simulink model "atrias_nmm_hardware"  (R2014b)
settings: Solver=ode4  StartTime=0.0  StopTime=inf  FixedStep=sample_time  RelTol=1e-3
undefined symbols (not defined in the file): A_lpf_dtau, B1_lpf_dtau, B2_lpf_dtau, boom_mount_angle, boom_pelvis_offset_angle, c, c_jointstop, contactThr, control_start_time, D12_T, d_y_boom_com_offset, d_y_boom_hip_offset, eref, fcut_contact, FmaxBFSH, FmaxGLU, FmaxHAM, FmaxHFL, FmaxRF, FmaxVAS, g, h_boom, HIP_MTR_MAX_CONT_TORQUE, initial_com_height, initial_dx, K, k_sea, kd_lateral, kd_phi12, kd_phi23, kp_lateral, kp_phi12, kp_phi23, l_boom_projected, L_distribution_switch, L_force_ctrl_switch, L_hip_trq_desired, L_knee_trq_desired, L_sea_input_switch, l_seg, L_stim_gain, L_stim_switch, l_yaw_center_to_pelvis, lambdaHip, lambdaKnee, lateral_offset, lateral_target_angle_left, lateral_target_angle_right, lateral_transition_force, loptBFSH, loptGLU, loptHAM, loptHFL, loptRF, loptVAS, Lphi12_des, Lphi23_des, lslackBFSH, lslackGLU, lslackHAM ... (+69)
libraries: simulink_extras x15, simulink x5, slrtlib x3
(part 2 of 9)

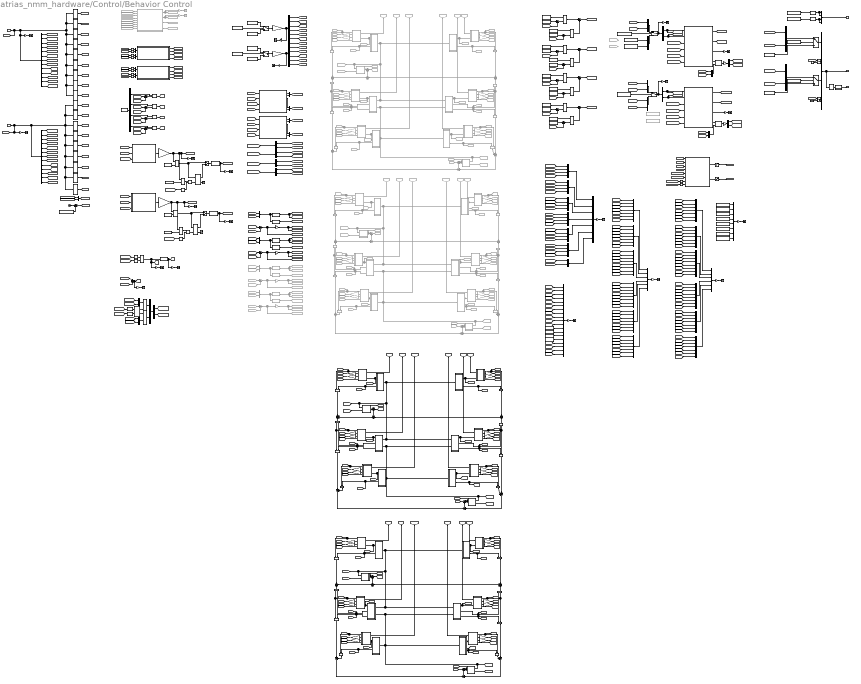
== system atrias_nmm_hardware/Control/Behavior Control ==
  note: Velocity Estimation
  note: Muscle Stimulation Input
  note: Leg/Spring Measurements
  note: Lateral Behavior
  note: Torque Commands
  note: Inputs
  note: q Order:
      |
      | backJointR
      | backGearR
      | frontJointR
      | frontGearR
      |
      | backJointL
      | backGearL
      | frontJointL
      | frontGearL
      |
      | latR
      | latL
      |
      | boomRoll
      | boomYaw
      | boomPitch
  note: Motor Order:
      |
      | backR
      | frontR
      | latR
      | backL
      | frontL
      | latL
  note: Muscle Geometry Input
  note: Atrias Knee/Splay Angles
  note: Estimate SEA Torque
  note: Estimate Leg Load and Contact
  note: Hip/Knee Torque Distribution
  note: Left Leg
  note: Neural Control Layer Interface
  note: Discrete Muscle Actuation Layer
  note: Body Mechanics Layer
      | Interface (Left Hip Joint)
  note: Body Mechanics Layer
      | Interface (Left Knee Joint)
  note: Right Leg
  note: Neural Control Layer Interface
  note: Body Mechanics Layer
      | Interface (Left Hip Joint)
  note: Body Mechanics Layer
      | Interface (Left Knee Joint)
  note: Estimate Flight/Escape
  note: Estimate GRFy
  note: Estimate Primary Leg Length/Angle
  note: Position Control
  note: Export Data
  note: Left Leg
  note: Neural Control Layer Interface
  note: Continuous Muscle Actuation Layer
  note: Body Mechanics Layer
      | Interface (Left Hip Joint)
  note: Body Mechanics Layer
      | Interface (Left Knee Joint)
  note: Right Leg
  note: Neural Control Layer Interface
  note: Body Mechanics Layer
      | Interface (Left Hip Joint)
  note: Body Mechanics Layer
      | Interface (Left Knee Joint)
  dq_cmu : Inport
  q_cmu : Inport  Port=2
  Clock : Clock
  Constant{,1,26,30,34,38} (6 alike) : Constant  Value=0
  Constant10 : Constant  Value=releaseThr
  Constant11 : Constant  Value=contactThr
  Constant12 : Constant  Value=releaseThr
  Constant13 : Constant  Commented=on  Value=L_knee_trq_desired
  Constant14 : Constant  Value=R_knee_trq_desired
  Constant15 : Constant  Value=R_distribution_switch
  Constant16 : Constant  Value=L_distribution_switch
  Constant17 : Constant  Value=R_sea_input_switch
  Constant18 : Constant  Value=L_sea_input_switch
  Constant19 : Constant  Value=[0;0]
  Constant2 : Constant  Value=control_start_time
  Constant20 : Constant  Value=[0;0]
  Constant21 : Constant  Value=R_hip_trq_desired
  Constant22 : Constant  Commented=on  Value=L_hip_trq_desired
  Constant23 : Constant  Value=k_sea
  Constant24 : Constant  Value=Lphi12_des
  Constant25 : Constant  Value=kp_phi12
  Constant27 : Constant  Value=kd_phi12
  Constant28 : Constant  Value=Lphi23_des
  Constant29 : Constant  Value=kp_phi23
  Constant3 : Constant  Value=LStim_Constant
  Constant31 : Constant  Value=kd_phi23
  Constant32 : Constant  Value=Rphi12_des
  Constant33 : Constant  Value=kp_phi12
  Constant35 : Constant  Value=kd_phi12
  Constant36 : Constant  Value=Rphi23_des
  Constant37 : Constant  Value=kp_phi23
  Constant39 : Constant  Value=kd_phi23
  Constant4 : Constant  Value=RStim_Constant
  Constant40 : Constant  Value=Lphi23_des
  Constant41 : Constant  Value=Lphi12_des
  Constant42 : Constant  Value=Rphi23_des
  Constant43 : Constant  Value=Rphi12_des
  Constant44 : Constant  Value=R_force_ctrl_switch
  Constant45 : Constant  Value=L_force_ctrl_switch
  Constant46 : Constant  Value=R_distribution_switch
  Constant47 : Constant  Value=L_distribution_switch
  Constant48 : Constant  Value=R_stim_switch
  Constant49 : Constant  Value=L_stim_switch
  Constant5 : Constant  Value=[0;0;0;0;0;0]
  Constant50 : Constant  Value=R_force_ctrl_switch
  Constant51 : Constant  Value=L_force_ctrl_switch
  Constant52 : Constant  Value=R_sea_input_switch
  Constant53 : Constant  Value=L_sea_input_switch
  Constant6 : Constant  Value=[0;0;0;0;0;0]
  Constant7 : Constant  Value=R_stim_switch
  Constant8 : Constant  Value=L_stim_switch
  Constant9 : Constant  Value=contactThr
  Data Type Conversion : DataTypeConversion  OutDataTypeStr=double
  Data Type Conversion1 : DataTypeConversion  OutDataTypeStr=double
  Data Type Conversion{2..5} (4 alike) : DataTypeConversion  OutDataTypeStr=boolean
  Demux{,1,3,14..19} (9 alike) : Demux  Outputs=2
  Demux11 : Demux  Outputs=6
  Demux12 : Demux  Outputs=13
  Demux13 : Demux  Outputs=13
  Demux2 : Demux  Outputs=6
  Demux4 : Demux
  Detect Increase : simulink/Logic and Bit Operations/Detect Increase  vinit=0.0  InputProcessing=Inherited  OutDataTypeStr=boolean
  From10 : From  Commented=on  GotoTag=Lphi12  TagVisibility=global
      settings: CloseFcn=tagdialog Close
  From116 : From  Commented=on  GotoTag=qBoomYaw
  From12 : From  Commented=on  GotoTag=Ldphi23  TagVisibility=global
      settings: CloseFcn=tagdialog Close
  From13 : From  Commented=on  GotoTag=RStimVAS  TagVisibility=global
      settings: CloseFcn=tagdialog Close
  From16 : From  Commented=on  GotoTag=Rdphi23  TagVisibility=global
      settings: CloseFcn=tagdialog Close
  From17 : From  Commented=on  GotoTag=Lphi23  TagVisibility=global
      settings: CloseFcn=tagdialog Close
  From19 : From  Commented=on  GotoTag=RStimRF  TagVisibility=global
      settings: CloseFcn=tagdialog Close
  From21 : From  Commented=on  GotoTag=LStimRF  TagVisibility=global
      settings: CloseFcn=tagdialog Close
  From22 : From  Commented=on  GotoTag=GRFy
  From23 : From  Commented=on  GotoTag=RStimHAM  TagVisibility=global
      settings: CloseFcn=tagdialog Close
  From24 : From  Commented=on  GotoTag=Ldphi12  TagVisibility=global
      settings: CloseFcn=tagdialog Close
  From25 : From  Commented=on  GotoTag=RStimHFL  TagVisibility=global
      settings: CloseFcn=tagdialog Close
  From26 : From  Commented=on  GotoTag=RStimGLU  TagVisibility=global
      settings: CloseFcn=tagdialog Close
  From260 : From  Commented=on  GotoTag=Lphi_thigh  TagVisibility=global
  From261 : From  Commented=on  GotoTag=Lphi_shin  TagVisibility=global
  From262 : From  Commented=on  GotoTag=Ldphi_thigh  TagVisibility=global
  From263 : From  Commented=on  GotoTag=Rphi_thigh  TagVisibility=global
  From264 : From  Commented=on  GotoTag=Rphi_shin  TagVisibility=global
  From265 : From  Commented=on  GotoTag=Rdphi_thigh  TagVisibility=global
  From266 : From  Commented=on  GotoTag=Rdphi_shin  TagVisibility=global
  From267 : From  Commented=on  GotoTag=Ldphi_shin  TagVisibility=global
  From28 : From  Commented=on  GotoTag=dqBoomYaw
  From29 : From  Commented=on  GotoTag=qBoomRoll
  From33 : From  Commented=on  GotoTag=RStimBFSH  TagVisibility=global
      settings: CloseFcn=tagdialog Close
  From34 : From  Commented=on  GotoTag=Rphi12  TagVisibility=global
      settings: CloseFcn=tagdialog Close
  From35 : From  Commented=on  GotoTag=LStimHAM  TagVisibility=global
      settings: CloseFcn=tagdialog Close
  From36 : From  Commented=on  GotoTag=Rdphi12  TagVisibility=global
      settings: CloseFcn=tagdialog Close
  From37 : From  Commented=on  GotoTag=LStimHFL  TagVisibility=global
      settings: CloseFcn=tagdialog Close
  From38 : From  Commented=on  GotoTag=LStimGLU  TagVisibility=global
      settings: CloseFcn=tagdialog Close
  From39 : From  Commented=on  GotoTag=LStimBFSH  TagVisibility=global
      settings: CloseFcn=tagdialog Close
  From40 : From  Commented=on  GotoTag=Rphi23  TagVisibility=global
      settings: CloseFcn=tagdialog Close
  From45 : From  Commented=on  GotoTag=TorsoPitch
  From50 : From  Commented=on  GotoTag=PrimaryLegAngle
  From51 : From  Commented=on  GotoTag=PrimaryLegLength
  From52 : From  Commented=on  GotoTag=dqBoomRoll
  From69 : From  Commented=on  GotoTag=RM23_pd  TagVisibility=global
  From70 : From  Commented=on  GotoTag=RM12_pd  TagVisibility=global
  From81 : From  Commented=on  GotoTag=escape
  From9 : From  Commented=on  GotoTag=LStimVAS  TagVisibility=global
      settings: CloseFcn=tagdialog Close
  GLU : Subsystem
  GLU Link : Subsystem  Commented=on
  GLU Link1 : Subsystem  Commented=on
  GLU Link2 : Subsystem
  GLU Link3 : Subsystem
  GLU1 : Subsystem
  GRFy : Gain
  Gain{,2,4..5} (4 alike) : Gain  Gain=-1
  Gain1 : Gain  Gain=R_stim_gain
  Gain3 : Gain  Gain=L_stim_gain
  Gain6 : Gain  Commented=on  Gain=-1
  Gain7 : Gain  Commented=on  Gain=-1
  Goto100 : Goto  Commented=on  GotoTag=RHipStop  TagVisibility=global
  Goto101 : Goto  Commented=on  GotoTag=RKneeStop  TagVisibility=global
  Goto102 : Goto  Commented=on  GotoTag=RLceHFL  TagVisibility=global
  Goto103 : Goto  Commented=on  GotoTag=RActRF  TagVisibility=global
  Goto104 : Goto  Commented=on  GotoTag=LFmRF  TagVisibility=global
  Goto105 : Goto  Commented=on  GotoTag=RActBFSH  TagVisibility=global
  Goto106 : Goto  Commented=on  GotoTag=RActVAS  TagVisibility=global
  Goto107 : Goto  Commented=on  GotoTag=RVceHAM  TagVisibility=global
  Goto108 : Goto  Commented=on  GotoTag=RrBFSH  TagVisibility=global
  Goto109 : Goto  Commented=on  GotoTag=RVceGLU  TagVisibility=global
  Goto110 : Goto  Commented=on  GotoTag=RLceGLU  TagVisibility=global
  Goto111 : Goto  Commented=on  GotoTag=RFmHFL  TagVisibility=global
  Goto112 : Goto  Commented=on  GotoTag=RVceVAS  TagVisibility=global
  Goto113 : Goto  Commented=on  GotoTag=LHipStop  TagVisibility=global
  Goto114 : Goto  Commented=on  GotoTag=LKneeStop  TagVisibility=global
  Goto115 : Goto  Commented=on  GotoTag=LLmtuBFSH  TagVisibility=global
  Goto116 : Goto  Commented=on  GotoTag=LActRF  TagVisibility=global
  Goto117 : Goto  Commented=on  GotoTag=LActBFSH  TagVisibility=global
  Goto124 : Goto  Commented=on  GotoTag=LFmBFSH  TagVisibility=global
  Goto126 : Goto  Commented=on  GotoTag=LVceHFL  TagVisibility=global
  Goto133 : Goto  Commented=on  GotoTag=Lphi_lower_splay  TagVisibility=global
  Goto134 : Goto  Commented=on  GotoTag=Ldphi_lower_splay  TagVisibility=global
  Goto135 : Goto  Commented=on  GotoTag=Lphi_back_knee  TagVisibility=global
  Goto136 : Goto  Commented=on  GotoTag=Ldphi_back_knee  TagVisibility=global
  Goto137 : Goto  Commented=on  GotoTag=Lphi_front_knee  TagVisibility=global
  Goto138 : Goto  Commented=on  GotoTag=Ldphi_front_knee  TagVisibility=global
  Goto139 : Goto  Commented=on  GotoTag=Rphi_lower_splay  TagVisibility=global
  Goto140 : Goto  Commented=on  GotoTag=Rdphi_lower_splay  TagVisibility=global
  Goto141 : Goto  Commented=on  GotoTag=Rphi_back_knee  TagVisibility=global
  Goto142 : Goto  Commented=on  GotoTag=Rdphi_back_knee  TagVisibility=global
  Goto143 : Goto  Commented=on  GotoTag=Rphi_front_knee  TagVisibility=global
  Goto144 : Goto  Commented=on  GotoTag=Rdphi_front_knee  TagVisibility=global
  Goto22 : Goto  Commented=on  GotoTag=LM12  TagVisibility=global
  Goto23 : Goto  Commented=on  GotoTag=RM12  TagVisibility=global
  Goto24 : Goto  Commented=on  GotoTag=LM23  TagVisibility=global
  Goto26 : Goto  Commented=on  GotoTag=dx_avg
  Goto27 : Goto  Commented=on  GotoTag=LLmtuVAS  TagVisibility=global
  Goto28 : Goto  Commented=on  GotoTag=RFmRF  TagVisibility=global
  Goto36 : Goto  Commented=on  GotoTag=LrHFL  TagVisibility=global
  Goto37 : Goto  Commented=on  GotoTag=LActHAM  TagVisibility=global
  Goto38 : Goto  Commented=on  GotoTag=LActGLU  TagVisibility=global
  Goto39 : Goto  Commented=on  GotoTag=LActHFL  TagVisibility=global
  Goto40 : Goto  Commented=on  GotoTag=LrHAMh  TagVisibility=global
  Goto41 : Goto  Commented=on  GotoTag=LrHAMk  TagVisibility=global
  Goto42 : Goto  Commented=on  GotoTag=LLceHAM  TagVisibility=global
  Goto43 : Goto  Commented=on  GotoTag=LrRFh  TagVisibility=global
  Goto44 : Goto  Commented=on  GotoTag=LrRFk  TagVisibility=global
  Goto45 : Goto  Commented=on  GotoTag=LLmtuRF  TagVisibility=global
  Goto46 : Goto  Commented=on  GotoTag=LrVAS  TagVisibility=global
  Goto47 : Goto  Commented=on  GotoTag=LLceRF  TagVisibility=global
  Goto48 : Goto  Commented=on  GotoTag=dy_avg
  Goto49 : Goto  Commented=on  GotoTag=tApex
  Goto50 : Goto  Commented=on  GotoTag=systemEnergy
  Goto51 : Goto  Commented=on  GotoTag=LVceBFSH  TagVisibility=global
  Goto52 : Goto  Commented=on  GotoTag=LLceBFSH  TagVisibility=global
  Goto53 : Goto  Commented=on  GotoTag=LLceVAS  TagVisibility=global
  Goto54 : Goto  Commented=on  GotoTag=LLmtuHFL  TagVisibility=global
  Goto56 : Goto  Commented=on  GotoTag=LFmGLU  TagVisibility=global
  Goto57 : Goto  Commented=on  GotoTag=LVceRF  TagVisibility=global
  Goto58 : Goto  Commented=on  GotoTag=LFmHAM  TagVisibility=global
  Goto59 : Goto  Commented=on  GotoTag=LFmVAS  TagVisibility=global
  Goto60 : Goto  Commented=on  GotoTag=RLmtuGLU  TagVisibility=global
  Goto61 : Goto  Commented=on  GotoTag=RLmtuHAM  TagVisibility=global
  Goto62 : Goto  Commented=on  GotoTag=LrGLU  TagVisibility=global
  Goto63 : Goto  Commented=on  GotoTag=RM23  TagVisibility=global
  Goto64 : Goto  Commented=on  GotoTag=RLmtuBFSH  TagVisibility=global
  Goto65 : Goto  Commented=on  GotoTag=RLmtuVAS  TagVisibility=global
  Goto66 : Goto  Commented=on  GotoTag=LLceHFL  TagVisibility=global
  Goto67 : Goto  Commented=on  GotoTag=RLmtuRF  TagVisibility=global
  Goto68 : Goto  Commented=on  GotoTag=LActVAS  TagVisibility=global
  Goto69 : Goto  Commented=on  GotoTag=LVceHAM  TagVisibility=global
  Goto70 : Goto  Commented=on  GotoTag=RFmBFSH  TagVisibility=global
  Goto71 : Goto  Commented=on  GotoTag=RVceHFL  TagVisibility=global
  Goto72 : Goto  Commented=on  GotoTag=RrHFL  TagVisibility=global
  Goto73 : Goto  Commented=on  GotoTag=RActHAM  TagVisibility=global
  Goto74 : Goto  Commented=on  GotoTag=RLmtuHFL  TagVisibility=global
  Goto75 : Goto  Commented=on  GotoTag=RActGLU  TagVisibility=global
  Goto76 : Goto  Commented=on  GotoTag=RActHFL  TagVisibility=global
  Goto77 : Goto  Commented=on  GotoTag=RrHAMh  TagVisibility=global
  Goto79 : Goto  Commented=on  GotoTag=RrHAMk  TagVisibility=global
  Goto80 : Goto  Commented=on  GotoTag=LLmtuGLU  TagVisibility=global
  Goto81 : Goto  Commented=on  GotoTag=RLceHAM  TagVisibility=global
  Goto82 : Goto  Commented=on  GotoTag=RrRFh  TagVisibility=global
  Goto83 : Goto  Commented=on  GotoTag=RrRFk  TagVisibility=global
  Goto84 : Goto  Commented=on  GotoTag=RrVAS  TagVisibility=global
  Goto85 : Goto  Commented=on  GotoTag=RLceRF  TagVisibility=global
  Goto86 : Goto  Commented=on  GotoTag=LVceGLU  TagVisibility=global
  Goto87 : Goto  Commented=on  GotoTag=LLceGLU  TagVisibility=global
  Goto88 : Goto  Commented=on  GotoTag=LFmHFL  TagVisibility=global
  Goto89 : Goto  Commented=on  GotoTag=RVceBFSH  TagVisibility=global
  Goto90 : Goto  Commented=on  GotoTag=LLmtuHAM  TagVisibility=global
  Goto91 : Goto  Commented=on  GotoTag=RLceBFSH  TagVisibility=global
  Goto92 : Goto  Commented=on  GotoTag=RLceVAS  TagVisibility=global
  Goto93 : Goto  Commented=on  GotoTag=LVceVAS  TagVisibility=global
  Goto94 : Goto  Commented=on  GotoTag=RFmGLU  TagVisibility=global
  Goto95 : Goto  Commented=on  GotoTag=RVceRF  TagVisibility=global
  Goto96 : Goto  Commented=on  GotoTag=RFmHAM  TagVisibility=global
  Goto97 : Goto  Commented=on  GotoTag=LrBFSH  TagVisibility=global
  Goto98 : Goto  Commented=on  GotoTag=RFmVAS  TagVisibility=global
  Goto99 : Goto  Commented=on  GotoTag=RrGLU  TagVisibility=global
  HAM : Subsystem
  HAM Link : Subsystem  Commented=on
  HAM Link1 : Subsystem  Commented=on
  HAM Link2 : Subsystem
  HAM Link3 : Subsystem
  HAM1 : Subsystem
  HFL : Subsystem
  HFL Link : Subsystem  Commented=on
  HFL Link1 : Subsystem  Commented=on
  HFL Link2 : Subsystem
  HFL Link3 : Subsystem
  HFL1 : Subsystem
  L BFSH : Subsystem  Commented=on
  L BFSH Link : Subsystem  Commented=on
  L BFSH Link1 : Subsystem  Commented=on
  L BFSH Link2 : Subsystem
  L BFSH Link3 : Subsystem
  L BFSH1 : Subsystem
  L BFSH2 : Subsystem
  L GLU : Subsystem  Commented=on
  L Geometry : Subsystem
  L HAM : Subsystem  Commented=on
  L HFL : Subsystem  Commented=on
  L HFL Muscle Spindles{,1,4..5} (4 alike) : Gain  Commented=on  Gain=1/loptHFL
  L HFL Muscle Spindles{10..11,14..15} (4 alike) : Gain  Gain=1/loptGLU
  L HFL Muscle Spindles{8..9,12..13} (4 alike) : Gain  Gain=1/loptHFL
  L HFL Muscle Spindles{2..3,6..7} (4 alike) : Gain  Commented=on  Gain=1/loptGLU
  L Hip Joint Limits : Subsystem  Commented=on
  L Hip Joint Limits1 : Subsystem  Commented=on
  L Hip Joint Limits2 : Subsystem
  L Hip Joint Limits3 : Subsystem
  L Knee Joint Limits : Subsystem  Commented=on
  L Knee Joint Limits1 : Subsystem  Commented=on
  L Knee Joint Limits2 : Subsystem
  L Knee Joint Limits3 : Subsystem
  L Leg Calculator : Subsystem
  L Leg Load : Subsystem
  L RF : Subsystem  Commented=on
  L RF Muscle Spindles{,1..3} (4 alike) : Gain  Commented=on  Gain=1/loptRF
  L RF Muscle Spindles{8..11} (4 alike) : Gain  Gain=1/loptRF
  L RF Muscle Spindles{12..15} (4 alike) : Gain  Gain=1/loptVAS
  L RF Muscle Spindles{4..7} (4 alike) : Gain  Commented=on  Gain=1/loptVAS
  L Torque : Subsystem
  L VAS : Subsystem  Commented=on
  LLoad : Gain
  L_Contact : Gain
  L_distribution_constraint_flag : Gain
  L_muscle_states : Gain
  L_stim : Gain
  L_tau_virt_des : Gain
  Lateral Control : MATLAB Function  TreatAsAtomicUnit=on
  Left Lateral Torque Saturation : Saturate  UpperLimit=max_torque_lateral  LowerLimit=-max_torque_lateral
      settings: AttributesFormatString=Top: %<UpperLimit>\nBottom: %<LowerLimit>
  Logical Operator : Logic  Operator=NOT  AllPortsSameDT=off  OutDataTypeStr=boolean
  Logical Operator1 : Logic  AllPortsSameDT=off  OutDataTypeStr=boolean
  Logical Operator2 : Logic  AllPortsSameDT=off  OutDataTypeStr=boolean
  Logical Operator3 : Logic  Operator=NOT  AllPortsSameDT=off  OutDataTypeStr=boolean
  Logical Operator4 : Logic  AllPortsSameDT=off  OutDataTypeStr=boolean
  Manual Switch : ManualSwitch
  Manual Switch1 : ManualSwitch
  Manual Switch2 : ManualSwitch  CurrentSetting=0
  Manual Switch3 : ManualSwitch  CurrentSetting=0
  Matrix Multiply : Product  Multiplication=Matrix(*)
  Matrix Multiply1 : Product  Multiplication=Matrix(*)
  Memory : Memory
  Memory1 : Memory
  Mux{,3,14,16,19,29,31..32} (8 alike) : Mux
  Mux{1..2,4..13,17..18,20..28} (23 alike) : Mux  Inputs=2
  Mux{15,33..34,36,39..42,46} (9 alike) : Mux  Inputs=7
  Mux35 : Mux  Inputs=6
  Mux{37..38,43..44,48} (5 alike) : Mux  Inputs=8
  Mux45 : Mux  Inputs=6
  Mux47 : Mux  Inputs=19
  Mux49 : Mux  Commented=on  Inputs=2
  Mux50 : Mux  Commented=on  Inputs=2
  Product{,1..3,10..11,13,16,24..29} (14 alike) : Product
  Product{4..9,12,14..15,17..23} (16 alike) : Product  Commented=on  RndMeth=Zero
  Product{30..45} (16 alike) : Product  RndMeth=Zero
  R BFSH : Subsystem  Commented=on
  R GLU : Subsystem  Commented=on
  R Geometry : Subsystem
  R HAM : Subsystem  Commented=on
  R HAM Muscle Spindles{1,3,6,14} (4 alike) : Gain  Commented=on  Gain=1/loptHAM
  R HAM Muscle Spindles{7..8,10,15} (4 alike) : Gain  Gain=1/loptBFSH
  R HAM Muscle Spindles{5,9,11,16} (4 alike) : Gain  Gain=1/loptHAM
  R HAM Muscle Spindles{2,4,12..13} (4 alike) : Gain  Commented=on  Gain=1/loptBFSH
  R HFL : Subsystem  Commented=on
  R Leg Calculator : Subsystem
  R Leg Load : Subsystem
  R RF : Subsystem  Commented=on
  R Torque : Subsystem
  R VAS : Subsystem  Commented=on
  RF : Subsystem
  RF Link : Subsystem  Commented=on
  RF Link1 : Subsystem  Commented=on
  RF Link2 : Subsystem
  RF Link3 : Subsystem
  RF1 : Subsystem
  RLoad : Gain
  R_Contact : Gain
  R_distribution_constraint_flag : Gain
  R_muscle_states : Gain
  R_stim : Gain
  R_tau_virt_des : Gain
  Relational Operator : RelationalOperator  OutDataTypeStr=boolean
  Relational Operator1 : RelationalOperator  Operator=<=  OutDataTypeStr=boolean
  Relational Operator2 : RelationalOperator  OutDataTypeStr=boolean
  Relational Operator3 : RelationalOperator  Operator=<=  OutDataTypeStr=boolean
  Right Lateral Torque Saturation : Saturate  UpperLimit=max_torque_lateral  LowerLimit=-max_torque_lateral
      settings: AttributesFormatString=Top: %<UpperLimit>\nBottom: %<LowerLimit>
  S-R Flip-Flop : simulink_extras/Flip Flops/S-R Flip-Flop  initial_condition=0
  S-R Flip-Flop1 : simulink_extras/Flip Flops/S-R Flip-Flop  initial_condition=0
  S-R Flip-Flop2 : simulink_extras/Flip Flops/S-R Flip-Flop  initial_condition=0
  Selector{,3,14..17,24..27} (10 alike) : Selector  InputPortWidth=2  Indices=[1]
  Selector1 : Selector  InputPortWidth=13  Indices=[10]
  Selector10 : Selector  InputPortWidth=13  Indices=[7 8]
  Selector11 : Selector  InputPortWidth=13  Indices=[9]
  Selector12 : Selector  InputPortWidth=13  Indices=[1 2]
  Selector13 : Selector  InputPortWidth=13  Indices=[3 4]
  Selector18 : Selector  InputPortWidth=13  Indices=[13]
  Selector2 : Selector  InputPortWidth=13  Indices=[5 6]
  Selector20 : Selector  InputPortWidth=13  Indices=[13]
  Selector21 : Selector  InputPortWidth=13  Indices=[11]
  Selector22 : Selector  InputPortWidth=13  Indices=[12]
  Selector23 : Selector  InputPortWidth=13  Indices=[11]
  Selector28 : Selector  InputPortWidth=13  Indices=[12]
  Selector33 : Selector  InputPortWidth=6  Indices=[1 2 4 5]
  Selector4 : Selector  InputPortWidth=13  Indices=[7 8]
  Selector5 : Selector  InputPortWidth=13  Indices=[9]
  Selector6 : Selector  InputPortWidth=13  Indices=[1 2]
  Selector7 : Selector  InputPortWidth=13  Indices=[3 4]
  Selector8 : Selector  InputPortWidth=13  Indices=[10]
  Selector9 : Selector  InputPortWidth=13  Indices=[5 6]
  Sum{,2,4,6,9,15,20,24,26..27,29..30,32..33,35} (15 alike) : Sum  Inputs=|+-
  Sum{1,7,12,16,18,22} (6 alike) : Sum  Commented=on  Inputs=|++
  Sum10 : Sum  Commented=on  Inputs=+-
  Sum{3,8,11,19} (4 alike) : Sum  Commented=on
  Sum13 : Sum  Commented=on  Inputs=++|
  Sum14 : Sum  Commented=on  Inputs=+-
  Sum17 : Sum  Commented=on  Inputs=++|
  Sum21 : Sum  Commented=on  Inputs=-+
  Sum{23,40,47,50,53} (5 alike) : Sum
  Sum{25,28,31,34,38,41,44,46,49,52} (10 alike) : Sum  Inputs=|++
  Sum36 : Sum  Commented=on  Inputs=|+-
  Sum37 : Sum  Commented=on  Inputs=|+-
  Sum39 : Sum  Inputs=+-
  Sum42 : Sum  Inputs=++|
  Sum43 : Sum  Inputs=+-
  Sum45 : Sum  Inputs=++|
  Sum48 : Sum  Inputs=-+
  Sum5 : Sum  Commented=on  Inputs=-+
  Sum51 : Sum  Inputs=-+
  Switch : Switch  Criteria=u2 ~= 0
  Switch1 : Switch  Criteria=u2 ~= 0
  Switch{2..5} (4 alike) : Switch  Criteria=u2 > Threshold
  Terminator : Terminator  Commented=on
  Terminator{1..4,6..19,23..26} (22 alike) : Terminator
  Terminator5 : Terminator  Commented=on
  VAS : Subsystem
  VAS Link : Subsystem  Commented=on
  VAS Link1 : Subsystem  Commented=on
  VAS Link2 : Subsystem
  VAS Link3 : Subsystem
  VAS1 : Subsystem
  Velocity Estimation : Subsystem  Commented=on
  "[N] to [%bw]" : Gain  Gain=1/(m_total_real*g)
  dq : Gain
  dtau_des : Subsystem
  dx_avg : Gain  Commented=on
  dy_avg : Gain  Commented=on
  escape : Gain
  flight : Gain
  knee angle : Fcn  Expr=pi-(u(1)-u(2))
  knee angle1 : Fcn  Expr=pi-(u(1)-u(2))
  knee angle2 : Fcn  Commented=on  Expr=pi-(u(1)-u(2))
  knee angle3 : Fcn  Commented=on  Expr=pi-(u(1)-u(2))
  manual_switches : Gain
  percent body weight : Gain  Gain=1/(m_total_real*g)
  q : Gain
  splay angle : Fcn  Expr=(u(1)-u(2))
  splay angle1 : Fcn  Expr=(u(1)-u(2))
  splay angle2 : Fcn  Commented=on  Expr=(u(1)-u(2))
  splay angle3 : Fcn  Commented=on  Expr=(u(1)-u(2))
  torques : Gain
  virtual_kinematics : Gain
  Motor Torque Command [Nm] x6 : Outport  OutputWhenDisabled=reset  InitialOutput=[0 0 0 0 0 0]
  SEA Torque Velocity Command [Nm] x4 : Outport  Port=2  OutputWhenDisabled=reset  InitialOutput=[0 0 0 0 0 0]
  Force / Position Control [1/0] x4 : Outport  Port=3  OutputWhenDisabled=reset  InitialOutput=[0 0 0 0 0 0]
  tag scope: GRFy=global, LActBFSH=global, LActGLU=global, LActHAM=global, LActHFL=global, LActRF=global, LActVAS=global, LFmBFSH=global, LFmGLU=global, LFmHAM=global, LFmHFL=global, LFmRF=global, LFmVAS=global, LFootCnt=global, LHipStop=global, LKneeStop=global, LLLoad=global, LLceBFSH=global, LLceGLU=global, LLceHAM=global, LLceHFL=global, LLceRF=global, LLceVAS=global, LLmtuBFSH=global, LLmtuGLU=global, LLmtuHAM=global, LLmtuHFL=global, LLmtuRF=global, LLmtuVAS=global, LM12=global, LM12_achieved=global, LM12_des=global, LM12_pd=global, LM23=global, LM23_achieved=global, LM23_des=global, LM23_pd=global, LStimBFSH=global, LStimGLU=global, LStimHAM=global, LStimHFL=global, LStimRF=global, LStimVAS=global, LVceBFSH=global, LVceGLU=global, LVceHAM=global, LVceHFL=global, LVceRF=global, LVceVAS=global, Ldgear_shin=global, Ldgear_thigh=global, Ldphi12=global, Ldphi23=global, Ldphi_Lat=global, Ldphi_back_knee=global, Ldphi_front_knee=global, Ldphi_lower_splay=global, Ldphi_shin=global, Ldphi_thigh=global, Lgear_shin=global, Lgear_thigh=global, Lphi12=global, Lphi12dphi12=global, Lphi23=global, Lphi23dphi23=global, Lphi_Lat=global, Lphi_back_knee=global, Lphi_front_knee=global, Lphi_lower_splay=global, Lphi_shin=global, Lphi_thigh=global, LrBFSH=global, LrGLU=global, LrHAMh=global, LrHAMk=global, LrHFL=global, LrRFh=global, LrRFk=global, LrVAS=global, Lshin_ctrl_trq=global, LtauB=global, LtauF=global, Lthigh_ctrl_trq=global, RActBFSH=global, RActGLU=global, RActHAM=global, RActHFL=global, RActRF=global, RActVAS=global, RFmBFSH=global, RFmGLU=global, RFmHAM=global, RFmHFL=global, RFmRF=global, RFmVAS=global, RFootCnt=global, RHipStop=global, RKneeStop=global, RLLoad=global, RLceBFSH=global, RLceGLU=global, RLceHAM=global, RLceHFL=global, RLceRF=global, RLceVAS=global, RLmtuBFSH=global, RLmtuGLU=global, RLmtuHAM=global, RLmtuHFL=global, RLmtuRF=global, RLmtuVAS=global, RM12=global, RM12_achieved=global, RM12_des=global, RM12_pd=global, RM23=global, RM23_achieved=global, RM23_des=global, RM23_pd=global, RStimBFSH=global, RStimGLU=global, RStimHAM=global, RStimHFL=global, RStimRF=global, RStimVAS=global, RVceBFSH=global, RVceGLU=global, RVceHAM=global, RVceHFL=global, RVceRF=global, RVceVAS=global, Rdgear_shin=global, Rdgear_thigh=global, Rdphi12=global, Rdphi23=global, Rdphi_Lat=global, Rdphi_back_knee=global, Rdphi_front_knee=global, Rdphi_lower_splay=global, Rdphi_shin=global, Rdphi_thigh=global, Rgear_shin=global, Rgear_thigh=global, Rphi12=global, Rphi12dphi12=global, Rphi23=global, Rphi23dphi23=global, Rphi_Lat=global, Rphi_back_knee=global, Rphi_front_knee=global, Rphi_lower_splay=global, Rphi_shin=global, Rphi_thigh=global, RrBFSH=global, RrGLU=global, RrHAMh=global, RrHAMk=global, RrHFL=global, RrRFh=global, RrRFk=global, RrVAS=global, Rshin_ctrl_trq=global, RtauB=global, RtauF=global, Rthigh_ctrl_trq=global, droll=global, dtheta=global, dyaw=global, escape=global, flight=global, roll=global, theta=global, yaw=global
  wires:
  Switch1/1 -> Mux/3
  Mux18/1 -> Switch1/1
  Constant19/1 -> Switch/3
  Mux17/1 -> Switch/1
  [Lthigh_ctrl_trq] -> Mux18/2
  [Lshin_ctrl_trq] -> Mux18/1
  [Rshin_ctrl_trq] -> Mux17/1
  [Rthigh_ctrl_trq] -> Mux17/2
  Manual Switch/1 -> Mux/4
  Manual Switch1/1 -> Mux/2
  Switch/1 -> Mux/1
  Constant18/1 -> Switch1/2
  Constant17/1 -> Switch/2
  Mux3/1 -> Force / Position Control [1/0] x4/1
  Mux7/1 -> [TorsoPitch]
  [dqBoomPitch] -> Mux7/2
  [qBoomPitch] -> Mux7/1
  Velocity Estimation/4(system_energy [J]) -> Goto50/1
  dy_avg/1 -> Terminator5/1
  Velocity Estimation/3(t_apex [s]) -> Goto49/1
  Velocity Estimation/2(dy_avg [m/s]) -> Goto48/1, dy_avg/1
  dx_avg/1 -> Terminator/1
  Velocity Estimation/1(dx_avg [m/s]) -> Goto26/1, dx_avg/1
  L Leg Calculator/4(w [m]) -> [LLegW]
  R Leg Calculator/4(w [m]) -> [RLegW]
  Selector26/1 -> Mux4/1
  Selector27/1 -> Mux4/2
  Selector25/1 -> Mux5/2
  Selector24/1 -> Mux5/1
  L Leg Calculator/3(Leg Splay [rad rad/s]) -> [LLegSplay]
  L Leg Calculator/2(Leg Angle [rad rad/s]) -> [LLegAngle]
  L Leg Calculator/1("Leg Length [m m/s] ") -> [LLegLength]
  Mux4/1 -> L Leg Calculator/2(Back [rad rad/s])
  Mux5/1 -> L Leg Calculator/1(Front [rad rad/s])
  [dqFrontL] -> Selector25/1
  [qFrontL] -> Selector24/1
  [dqBackL] -> Selector27/1
  [qBackL] -> Selector26/1
  Selector23/1 -> [qBoomRoll]
  Selector21/1 -> [dqBoomRoll]
  Selector22/1 -> [dqBoomYaw]
  Selector20/1 -> [dqBoomPitch]
  Selector18/1 -> [qBoomPitch]
  Selector16/1 -> Mux1/1
  Selector17/1 -> Mux1/2
  Selector15/1 -> Mux2/2
  Selector14/1 -> Mux2/1
  [tauLatL] -> Manual Switch/1
  [tauLatR] -> Manual Switch1/1
  R Leg Calculator/3(Leg Splay [rad rad/s]) -> [RLegSplay]
  R Leg Calculator/2(Leg Angle [rad rad/s]) -> [RLegAngle]
  R Leg Calculator/1("Leg Length [m m/s] ") -> [RLegLength]
  Mux1/1 -> R Leg Calculator/2(Back [rad rad/s])
  Mux2/1 -> R Leg Calculator/1(Front [rad rad/s])
  [dqFrontR] -> Selector15/1
  [qFrontR] -> Selector14/1
  [dqBackR] -> Selector17/1
  [qBackR] -> Selector16/1
  Selector10/1 -> [dqFrontL]
  Selector9/1 -> [dqBackL]
  Selector13/1 -> [dqFrontR]
  Selector12/1 -> [dqBackR]
  Selector11/1 -> [dqLatR]
  Selector8/1 -> [dqLatL]
  Constant/1 -> Manual Switch/2
  Constant1/1 -> Manual Switch1/2
  Clock/1 -> Sum/1
  Constant2/1 -> Sum/2
  Selector5/1 -> [qLatR]
  Selector1/1 -> [qLatL]
  Selector6/1 -> [qBackR]
  Selector7/1 -> [qFrontR]
  Selector2/1 -> [qBackL]
  Selector4/1 -> [qFrontL]
  Sum/1 -> [controlClock]
  Lateral Control/1(tau_r) -> Right Lateral Torque Saturation/1
  Lateral Control/2(tau_l) -> Left Lateral Torque Saturation/1
  Right Lateral Torque Saturation/1 -> [tauLatR]
  Left Lateral Torque Saturation/1 -> [tauLatL]
  Selector33/1 -> dtau_des/1(x)
  dtau_des/1(dx/dt) -> SEA Torque Velocity Command [Nm] x4/1
  Mux/1 -> Selector33/1, Motor Torque Command [Nm] x6/1
  [dqLatR] -> Lateral Control/2(dqLateralR)
  [qLatR] -> Lateral Control/1(qLateralR)
  [dqLatL] -> Lateral Control/4(dqLateralL)
  [qLatL] -> Lateral Control/3(qLateralL)
  [RLegLength] -> Selector/1
  [LLegLength] -> Selector3/1
  [RLegMeasuredForce] -> Lateral Control/5(F_leg_R)
  [LLegMeasuredForce] -> Lateral Control/6(F_leg_L)
  Selector/1 -> Lateral Control/7(L_leg_R)
  Selector3/1 -> Lateral Control/8(L_leg_L)
  From29/1 -> Velocity Estimation/1(qRoll [rad])
  From52/1 -> Velocity Estimation/2(dqRoll [rad/s])
  From45/1 -> Velocity Estimation/3(Torso Pitch [rad rad/s])
  From116/1 -> Velocity Estimation/4(qYaw [rad])
  From28/1 -> Velocity Estimation/5(dqYaw [rad/s])
  From22/1 -> Velocity Estimation/7(GRFy [body weight])
  From81/1 -> Velocity Estimation/6(escape [1/0])
  From51/1 -> Velocity Estimation/8(Primary Leg Length [m m/s])
  From50/1 -> Velocity Estimation/9(Primary Leg Angle [rad rad/s])
  Selector28/1 -> [qBoomYaw]
  Constant3/1 -> Switch3/1
  Demux2/1 -> [LStimHFL]
  Demux2/2 -> [LStimGLU]
  Demux2/3 -> [LStimHAM]
  Demux2/4 -> [LStimRF]
  Demux2/5 -> [LStimVAS]
  Demux2/6 -> [LStimBFSH]
  Constant4/1 -> Switch2/1
  Demux11/1 -> [RStimHFL]
  Demux11/2 -> [RStimGLU]
  Demux11/3 -> [RStimHAM]
  Demux11/4 -> [RStimRF]
  Demux11/5 -> [RStimVAS]
  Demux11/6 -> [RStimBFSH]
  Constant5/1 -> Switch2/3
  Constant6/1 -> Switch3/3
  Constant7/1 -> Switch2/2
  Constant8/1 -> Switch3/2
  Demux12/1 -> [Rphi_shin]
  Demux12/2 -> [Rgear_shin]
  Demux12/3 -> [Rphi_thigh]
  Demux12/4 -> [Rgear_thigh]
  Demux12/5 -> [Lphi_shin]
  Demux12/6 -> [Lgear_shin]
  Demux12/7 -> [Lphi_thigh]
  Demux12/8 -> [Lgear_thigh]
  Demux12/9 -> [Rphi_Lat]
  Demux12/10 -> [Lphi_Lat]
  Demux12/11 -> [roll]
  Demux12/12 -> [yaw]
  Demux12/13 -> [theta]
  q_cmu/1 -> q/1, Demux12/1, Selector1/1, Selector23/1, Selector28/1, Selector18/1, Selector5/1, Selector4/1, Selector2/1, Selector7/1, Selector6/1, [qCMU]
  dq_cmu/1 -> Demux13/1, Selector10/1, Selector11/1, Selector8/1, Selector21/1, Selector22/1, Selector20/1, Selector9/1, Selector13/1, Selector12/1, [dqCMU], dq/1
  Demux13/13 -> [dtheta]
  Demux13/8 -> [Ldgear_thigh]
  Demux13/10 -> [Ldphi_Lat]
  Demux13/6 -> [Ldgear_shin]
  Demux13/9 -> [Rdphi_Lat]
  Demux13/11 -> [droll]
  Demux13/12 -> [dyaw]
  Demux13/4 -> [Rdgear_thigh]
  Demux13/5 -> [Ldphi_shin]
  Demux13/7 -> [Ldphi_thigh]
  Demux13/1 -> [Rdphi_shin]
  Demux13/3 -> [Rdphi_thigh]
  Demux13/2 -> [Rdgear_shin]
  [Lphi_front_knee] -> L Leg Load/3(phi_12 [rad])
  L Leg Load/1(Leg Load [N]) -> "[N] to [%bw]"/1
  [LtauF] -> L Leg Load/1(tau_F [Nm])
  [LtauB] -> L Leg Load/2(tau_B [Nm])
  [Lphi_front_knee] -> L Torque/5(phi12 [rad])
  [Lphi23dphi23] -> L Torque/4(v23dv23 [rad,rad/s])
  [Lphi_thigh] -> L Torque/6(phi23 [rad])
  [Lphi12dphi12] -> L Torque/3("v12dv12 [rad, rad/s]")
  Matrix Multiply/1 -> Gain/1
  L Torque/4(Jinv [2x2]) -> Matrix Multiply/1
  [Lgear_shin] -> Sum6/1
  Sum6/1 -> Product10/2
  [Lphi_shin] -> Sum6/2
  [Lgear_thigh] -> Sum2/1
  Sum2/1 -> Product11/2
  [Lphi_thigh] -> Sum2/2
  Mux20/1 -> splay angle/1, knee angle/1
  [Lgear_thigh] -> Mux20/2
  [Lgear_shin] -> Mux20/1
  knee angle/1 -> [Lphi_back_knee], [Lphi_front_knee]
  [Ldgear_thigh] -> Sum4/2
  [Ldgear_shin] -> Sum4/1
  Sum4/1 -> Gain2/1, [Ldphi_lower_splay]
  Gain2/1 -> [Ldphi_back_knee], [Ldphi_front_knee]
  splay angle/1 -> [Lphi_lower_splay]
  Relational Operator/1 -> S-R Flip-Flop/1, Manual Switch2/1
  Constant9/1 -> Relational Operator/2
  S-R Flip-Flop/1 -> Manual Switch2/2
  S-R Flip-Flop/2 -> Terminator1/1
  Logical Operator1/1 -> S-R Flip-Flop/2
  [RFootCnt] -> Memory/1
  Constant10/1 -> Relational Operator1/2
  Relational Operator1/1 -> Logical Operator1/1
  Memory/1 -> Logical Operator1/2
  Mux21/1 -> Matrix Multiply/2
  [LtauF] -> Mux21/1
  [LtauB] -> Mux21/2
  Demux14/2 -> [LM23_achieved]
  Demux14/1 -> [LM12_achieved]
  Data Type Conversion/1 -> L_Contact/1, [LFootCnt]
  Manual Switch2/1 -> Data Type Conversion/1
  [Ldphi_front_knee] -> L Geometry/3(dphi12 [rad])
  [Ldgear_thigh] -> L Geometry/4(dphi23 [rad])
  [Lgear_thigh] -> L Geometry/2(phi23 [rad])
  [Lphi_front_knee] -> L Geometry/1(phi12 [rad])
  L Geometry/3(dv12 [rad/s]) -> Mux23/2
  L Geometry/4(dv23 [rad/s]) -> Mux22/2
  Mux23/1 -> [Lphi12dphi12]
  Mux22/1 -> [Lphi23dphi23]
  L Geometry/1(v12 [rad]) -> Mux23/1
  L Geometry/2(v23 [rad]) -> Mux22/1
  [Lphi12dphi12] -> Demux15/1
  Demux15/1 -> [Lphi12]
  Demux15/2 -> [Ldphi12]
  [Lphi23dphi23] -> Demux16/1
  Demux16/1 -> [Lphi23]
  Demux16/2 -> [Ldphi23]
  [Rphi_front_knee] -> R Leg Load/3(phi_12 [rad])
  R Leg Load/1(Leg Load [N]) -> percent body weight/1
  [RtauF] -> R Leg Load/1(tau_F [Nm])
  [RtauB] -> R Leg Load/2(tau_B [Nm])
  Mux24/1 -> splay angle1/1, knee angle1/1
  [Rgear_thigh] -> Mux24/2
  [Rgear_shin] -> Mux24/1
  knee angle1/1 -> [Rphi_back_knee], [Rphi_front_knee]
  [Rdgear_thigh] -> Sum15/2
  [Rdgear_shin] -> Sum15/1
  Sum15/1 -> [Rdphi_lower_splay], Gain5/1
  Gain5/1 -> [Rdphi_back_knee], [Rdphi_front_knee]
  splay angle1/1 -> [Rphi_lower_splay]
  [Rgear_shin] -> Sum20/1
  Sum20/1 -> Product2/2
  [Rphi_shin] -> Sum20/2
  [Rgear_thigh] -> Sum9/1
  Sum9/1 -> Product3/2
  [Rphi_thigh] -> Sum9/2
  Relational Operator2/1 -> S-R Flip-Flop1/1, Manual Switch3/1
  Constant11/1 -> Relational Operator2/2
  S-R Flip-Flop1/1 -> Manual Switch3/2
  S-R Flip-Flop1/2 -> Terminator3/1
  Logical Operator2/1 -> S-R Flip-Flop1/2
  [LFootCnt] -> Memory1/1
  Constant12/1 -> Relational Operator3/2
  Relational Operator3/1 -> Logical Operator2/1
  Memory1/1 -> Logical Operator2/2
  Manual Switch3/1 -> Data Type Conversion1/1
  [Rdphi_front_knee] -> R Geometry/3(dphi12 [rad])
  [Rdgear_thigh] -> R Geometry/4(dphi23 [rad])
  [Rgear_thigh] -> R Geometry/2(phi23 [rad])
  [Rphi_front_knee] -> R Geometry/1(phi12 [rad])
  R Geometry/1(v12 [rad]) -> Mux27/1
  R Geometry/3(dv12 [rad/s]) -> Mux27/2
  R Geometry/4(dv23 [rad/s]) -> Mux26/2
  Mux27/1 -> [Rphi12dphi12]
  Mux26/1 -> [Rphi23dphi23]
  R Geometry/2(v23 [rad]) -> Mux26/1
  [Rphi12dphi12] -> Demux18/1
  Demux18/1 -> [Rphi12]
  Demux18/2 -> [Rdphi12]
  [Rphi23dphi23] -> Demux19/1
  Demux19/1 -> [Rphi23]
  Demux19/2 -> [Rdphi23]
  [Rphi12dphi12] -> R Torque/3("v12dv12 [rad, rad/s]")
  [Rphi23dphi23] -> R Torque/4(v23dv23 [rad,rad/s])
  [Rphi_front_knee] -> R Torque/5(phi12 [rad])
  [Rphi_thigh] -> R Torque/6(phi23 [rad])
  Matrix Multiply1/1 -> Gain4/1
  R Torque/4(Jinv [2x2]) -> Matrix Multiply1/1
  Mux25/1 -> Matrix Multiply1/2
  [RtauF] -> Mux25/1
  [RtauB] -> Mux25/2
  Demux17/2 -> [RM23_achieved]
  Demux17/1 -> [RM12_achieved]
  Mux6/1 -> Switch4/1
  Constant15/1 -> Switch4/2
  [RM12] -> Mux6/1
  [RM23] -> Mux6/2
  Demux/1 -> [RM12_des], R Torque/1(tau12_des [Nm])
  Demux/2 -> [RM23_des], R Torque/2(tau23_des [Nm])
  Mux8/1 -> Switch5/1
  Constant16/1 -> Switch5/2
  [LM12] -> Mux8/1
  [LM23] -> Mux8/2
  Constant20/1 -> Switch1/3
  Mux9/1 -> Switch4/3
  Constant14/1 -> Mux9/1
  Constant21/1 -> Mux9/2
  Mux10/1 -> Switch5/3
  From10/1 -> L Knee Joint Limits/1(phi [rad]1), VAS Link/1(phi23 [rad]), RF Link/2(phi23 [rad]), HAM Link/2(phi23 [rad]), L BFSH Link/1(phi23 [rad])
  From35/1 -> L HAM/1(STIM)
  L HAM/1(Fmtc) -> Product9/1, Product8/1, Goto58/1
  L HAM/2(Lce) -> R HAM Muscle Spindles1/1
  L HFL/1(Fmtc) -> Product7/2, Goto88/1
  L HFL/2(Lce) -> L HFL Muscle Spindles/1
  From37/1 -> L HFL/1(STIM)
  L GLU/1(Fmtc) -> Product6/1, Goto56/1
  From38/1 -> L GLU/1(STIM)
  Sum16/1 -> Goto24/1
  From24/1 -> L Knee Joint Limits/2(dphi [rad/s]1)
  VAS Link/1(lmtu [m]) -> Goto27/1, L VAS/2(lmtc [m])
  HAM Link/1(lmtu [m]) -> Goto90/1, L HAM/2(lmtc [m])
  HAM Link/2(lever34 [m]) -> Product8/2, Goto40/1
  HAM Link/3(lever23 [m]) -> Product9/2, Goto41/1
  Sum3/1 -> Sum14/1
  From17/1 -> L Hip Joint Limits/1(phi [rad]1), HFL Link/1(phi34 [rad]), GLU Link/1(phi34 [rad]), RF Link/1(phi34 [rad]), HAM Link/1(phi34 [rad])
  L VAS/4(A) -> Goto68/1
  L VAS/1(Fmtc) -> Product4/2, Goto59/1
  Sum1/1 -> Goto22/1
  L Knee Joint Limits/1(M_stop [Nm]1) -> Sum1/1, Goto114/1
  Sum5/1 -> Sum1/2
  VAS Link/2(lever [m]) -> Goto46/1, Product4/1
  Sum22/1 -> Sum5/1
  L HAM/4(A) -> Goto37/1
  Product8/1 -> Sum3/2
  Product6/1 -> Sum3/1
  GLU Link/1(lmtu [m]) -> Goto80/1, L GLU/2(lmtc [m])
  GLU Link/2(lever [m]) -> Product6/2, Goto62/1
  L GLU/4(A) -> Goto38/1
  From12/1 -> L Hip Joint Limits/2(dphi [rad/s]1)
  L Hip Joint Limits/1(M_stop [Nm]1) -> Goto113/1, Sum16/1
  Sum14/1 -> Sum16/2
  HFL Link/1(lmtu [m]) -> Goto54/1, L HFL/2(lmtc [m])
  L HFL/4(A) -> Goto39/1
  HFL Link/2(lever [m]) -> Product7/1, Goto36/1
  From9/1 -> L VAS/1(STIM)
  L GLU/2(Lce) -> L HFL Muscle Spindles3/1
  L GLU/3(Vce) -> L HFL Muscle Spindles2/1
  L HAM/3(Vce) -> R HAM Muscle Spindles6/1
  L VAS/3(Vce) -> L RF Muscle Spindles6/1
  L VAS/2(Lce) -> L RF Muscle Spindles4/1
  L HFL/3(Vce) -> L HFL Muscle Spindles1/1
  L RF/4(A) -> Goto116/1
  L RF/3(Vce) -> L RF Muscle Spindles2/1
  L RF/2(Lce) -> L RF Muscle Spindles/1
  RF Link/1(lmtu [m]) -> Goto45/1, L RF/2(lmtc [m])
  RF Link/2(lever34 [m]) -> Product5/1, Goto43/1
  RF Link/3(lever23 [m]) -> Product15/1, Goto44/1
  From21/1 -> L RF/1(STIM)
  Product7/1 -> Sum11/1
  Product5/1 -> Sum11/2
  Product15/1 -> Sum17/2
  Sum17/1 -> Sum5/2
  Product4/1 -> Sum17/1
  From39/1 -> L BFSH/1(STIM)
  L BFSH Link/1(lmtu [m]) -> Goto115/1, L BFSH/2(lmtc [m])
  L BFSH Link/2(lever [m]) -> Goto97/1, Product20/2
  L BFSH/4(A) -> Goto117/1
  L BFSH/2(Lce) -> R HAM Muscle Spindles4/1
  L BFSH/3(Vce) -> R HAM Muscle Spindles2/1
  Product20/1 -> Sum22/2
  Product9/1 -> Sum22/1
  L HFL Muscle Spindles1/1 -> Goto126/1
  L HFL Muscle Spindles2/1 -> Goto86/1
  L HFL Muscle Spindles3/1 -> Goto87/1
  L RF Muscle Spindles6/1 -> Goto93/1
  L RF/1(Fmtc) -> Product5/2, Product15/2, Goto104/1
  L BFSH/1(Fmtc) -> Product20/1, Goto124/1
  L HFL Muscle Spindles/1 -> Goto66/1
  R HAM Muscle Spindles1/1 -> Goto42/1
  R HAM Muscle Spindles6/1 -> Goto69/1
  L RF Muscle Spindles/1 -> Goto47/1
  L RF Muscle Spindles2/1 -> Goto57/1
  R HAM Muscle Spindles4/1 -> Goto52/1
  R HAM Muscle Spindles2/1 -> Goto51/1
  L RF Muscle Spindles4/1 -> Goto53/1
  From34/1 -> L Knee Joint Limits1/1(phi [rad]1), VAS Link1/1(phi23 [rad]), HAM Link1/2(phi23 [rad]), RF Link1/2(phi23 [rad]), L BFSH Link1/1(phi23 [rad])
  From23/1 -> R HAM/1(STIM)
  R HAM/1(Fmtc) -> Product23/1, Product22/1, Goto96/1
  R HAM/2(Lce) -> R HAM Muscle Spindles3/1
  R HFL/1(Fmtc) -> Product21/2, Goto111/1
  R HFL/2(Lce) -> L HFL Muscle Spindles4/1
  From25/1 -> R HFL/1(STIM)
  R GLU/1(Fmtc) -> Product19/1, Goto94/1
  From26/1 -> R GLU/1(STIM)
  Sum12/1 -> Goto63/1
  From36/1 -> L Knee Joint Limits1/2(dphi [rad/s]1)
  VAS Link1/1(lmtu [m]) -> Goto65/1, R VAS/2(lmtc [m])
  HAM Link1/1(lmtu [m]) -> Goto61/1, R HAM/2(lmtc [m])
  HAM Link1/2(lever34 [m]) -> Product22/2, Goto77/1
  HAM Link1/3(lever23 [m]) -> Product23/2, Goto79/1
  Sum19/1 -> Sum10/1
  From40/1 -> L Hip Joint Limits1/1(phi [rad]1), HFL Link1/1(phi34 [rad]), GLU Link1/1(phi34 [rad]), RF Link1/1(phi34 [rad]), HAM Link1/1(phi34 [rad])
  R VAS/4(A) -> Goto106/1
  R VAS/1(Fmtc) -> Product17/2, Goto98/1
  Sum7/1 -> Goto23/1
  L Knee Joint Limits1/1(M_stop [Nm]1) -> Sum7/1, Goto101/1
  Sum21/1 -> Sum7/2
  VAS Link1/2(lever [m]) -> Goto84/1, Product17/1
  Sum18/1 -> Sum21/1
  R HAM/4(A) -> Goto73/1
  Product22/1 -> Sum19/2
  Product19/1 -> Sum19/1
  GLU Link1/1(lmtu [m]) -> Goto60/1, R GLU/2(lmtc [m])
  GLU Link1/2(lever [m]) -> Product19/2, Goto99/1
  R GLU/4(A) -> Goto75/1
  From16/1 -> L Hip Joint Limits1/2(dphi [rad/s]1)
  L Hip Joint Limits1/1(M_stop [Nm]1) -> Goto100/1, Sum12/1
  Sum10/1 -> Sum12/2
  HFL Link1/1(lmtu [m]) -> Goto74/1, R HFL/2(lmtc [m])
  R HFL/4(A) -> Goto76/1
  HFL Link1/2(lever [m]) -> Product21/1, Goto72/1
  From13/1 -> R VAS/1(STIM)
  R GLU/2(Lce) -> L HFL Muscle Spindles7/1
  R GLU/3(Vce) -> L HFL Muscle Spindles6/1
  R HAM/3(Vce) -> R HAM Muscle Spindles14/1
  R VAS/3(Vce) -> L RF Muscle Spindles7/1
  R VAS/2(Lce) -> L RF Muscle Spindles5/1
  R HFL/3(Vce) -> L HFL Muscle Spindles5/1
  R RF/4(A) -> Goto103/1
  R RF/3(Vce) -> L RF Muscle Spindles3/1
  R RF/2(Lce) -> L RF Muscle Spindles1/1
  RF Link1/1(lmtu [m]) -> Goto67/1, R RF/2(lmtc [m])
  RF Link1/2(lever34 [m]) -> Product18/1, Goto82/1
  RF Link1/3(lever23 [m]) -> Goto83/1, Product12/1
  From19/1 -> R RF/1(STIM)
  Sum8/1 -> Sum10/2
  Product21/1 -> Sum8/1
  Product18/1 -> Sum8/2
  Product12/1 -> Sum13/2
  Sum13/1 -> Sum21/2
  Product17/1 -> Sum13/1
  From33/1 -> R BFSH/1(STIM)
  L BFSH Link1/1(lmtu [m]) -> Goto64/1, R BFSH/2(lmtc [m])
  L BFSH Link1/2(lever [m]) -> Goto108/1, Product14/2
  R BFSH/4(A) -> Goto105/1
  R BFSH/2(Lce) -> R HAM Muscle Spindles13/1
  R BFSH/3(Vce) -> R HAM Muscle Spindles12/1
  Product14/1 -> Sum18/2
  Product23/1 -> Sum18/1
  L HFL Muscle Spindles5/1 -> Goto71/1
  L HFL Muscle Spindles6/1 -> Goto109/1
  L HFL Muscle Spindles7/1 -> Goto110/1
  L RF Muscle Spindles7/1 -> Goto112/1
  R RF/1(Fmtc) -> Product18/2, Product12/2, Goto28/1
  R BFSH/1(Fmtc) -> Product14/1, Goto70/1
  L HFL Muscle Spindles4/1 -> Goto102/1
  R HAM Muscle Spindles3/1 -> Goto81/1
  R HAM Muscle Spindles14/1 -> Goto107/1
  L RF Muscle Spindles1/1 -> Goto85/1
  L RF Muscle Spindles3/1 -> Goto95/1
  R HAM Muscle Spindles13/1 -> Goto91/1
  R HAM Muscle Spindles12/1 -> Goto89/1
  L RF Muscle Spindles5/1 -> Goto92/1
  Sum11/1 -> Sum14/2
  [RFootCnt] -> Logical Operator/1
  [LFootCnt] -> Logical Operator3/1
  Logical Operator/1 -> Logical Operator4/1
  Logical Operator3/1 -> Logical Operator4/2
  Detect Increase/1 -> escape/1, [escape]
  [RLLoad] -> Sum23/1
  [LLLoad] -> Sum23/2
  Sum23/1 -> GRFy/1, [GRFy]
  [RLegLength] -> Mux11/1
  [RLegAngle] -> Mux11/2
  [LLegLength] -> Mux12/1
  [LLegAngle] -> Mux12/2
  [RFootCnt] -> Data Type Conversion4/1
  [LFootCnt] -> Data Type Conversion5/1
  S-R Flip-Flop2/2 -> Product1/1
  S-R Flip-Flop2/1 -> Product/2
  Mux11/1 -> Product/1
  Mux12/1 -> Product1/2
  Product/1 -> Mux13/1
  Product1/1 -> Mux13/2
  Mux13/1 -> Demux3/1
  Demux3/1 -> [PrimaryLegLength]
  Demux3/2 -> [PrimaryLegAngle]
  Constant23/1 -> Demux4/1
  Demux4/1 -> Product2/1
  Demux4/2 -> Product3/1
  Demux4/3 -> Product10/1
  Demux4/4 -> Product11/1
  L_Contact/1 -> Terminator2/1
  Data Type Conversion1/1 -> R_Contact/1, [RFootCnt]
  R_Contact/1 -> Terminator4/1
  Logical Operator4/1 -> Detect Increase/1, [flight], flight/1
  flight/1 -> Terminator6/1
  percent body weight/1 -> Relational Operator3/1, RLoad/1, [RLLoad], Relational Operator2/1
  RLoad/1 -> Terminator7/1
  "[N] to [%bw]"/1 -> Relational Operator/1, Relational Operator1/1, LLoad/1, [LLLoad]
  LLoad/1 -> Terminator8/1
  Switch2/1 -> Gain1/1
  R_stim/1 -> Terminator9/1
  Switch3/1 -> Gain3/1
  L_stim/1 -> Terminator10/1
  Switch4/1 -> R_tau_virt_des/1, Demux/1
  R_tau_virt_des/1 -> Terminator11/1
  Switch5/1 -> L_tau_virt_des/1, Demux1/1
  L_tau_virt_des/1 -> Terminator12/1
  Product2/1 -> [RtauB]
  Product3/1 -> [RtauF]
  Product10/1 -> [LtauB]
  Product11/1 -> [LtauF]
  Gain4/1 -> Demux17/1
  Gain/1 -> Demux14/1
  L Torque/2(tau_B [Nm]) -> [Lshin_ctrl_trq]
  L Torque/1(tau_F [Nm]) -> [Lthigh_ctrl_trq]
  R Torque/2(tau_B [Nm]) -> [Rshin_ctrl_trq]
  R Torque/1(tau_F [Nm]) -> [Rthigh_ctrl_trq]
  Gain1/1 -> R_stim/1, Demux11/1
  Gain3/1 -> L_stim/1, Demux2/1
  Data Type Conversion2/1 -> Mux3/1, Mux3/2
  Data Type Conversion3/1 -> Mux3/3, Mux3/4
  Data Type Conversion4/1 -> S-R Flip-Flop2/1
  Data Type Conversion5/1 -> S-R Flip-Flop2/2
  R Torque/3(constraint flag [0/1]) -> R_distribution_constraint_flag/1
  R_distribution_constraint_flag/1 -> Terminator23/1
  L Torque/3(constraint_flag [0/1]) -> L_distribution_constraint_flag/1
  L_distribution_constraint_flag/1 -> Terminator24/1
  Constant24/1 -> Sum24/1
  [Lphi12] -> Sum24/2
  Constant25/1 -> Product13/1
  Sum24/1 -> Product13/2
  Product13/1 -> Sum25/1
  Constant26/1 -> Sum26/1
  [Ldphi12] -> Sum26/2
  Constant27/1 -> Product16/1
  Sum26/1 -> Product16/2
  Product16/1 -> Sum25/2
  Sum25/1 -> [LM12_pd]
  Constant28/1 -> Sum27/1
  [Lphi23] -> Sum27/2
  Constant29/1 -> Product24/1
  Sum27/1 -> Product24/2
  Product24/1 -> Sum28/1
  Constant30/1 -> Sum29/1
  [Ldphi23] -> Sum29/2
  Constant31/1 -> Product25/1
  Sum29/1 -> Product25/2
  Product25/1 -> Sum28/2
  Sum28/1 -> [LM23_pd]
  [LM12_pd] -> Mux10/1
  [LM23_pd] -> Mux10/2
  Constant32/1 -> Sum30/1
  [Rphi12] -> Sum30/2
  Sum30/1 -> Product26/2
  Product26/1 -> Sum31/1
  Constant34/1 -> Sum32/1
  [Rdphi12] -> Sum32/2
  Constant35/1 -> Product27/1
  Sum32/1 -> Product27/2
  Product27/1 -> Sum31/2
  Sum31/1 -> [RM12_pd]
  Constant36/1 -> Sum33/1
  [Rphi23] -> Sum33/2
  Constant37/1 -> Product28/1
  Sum33/1 -> Product28/2
  Product28/1 -> Sum34/1
  Constant38/1 -> Sum35/1
  [Rdphi23] -> Sum35/2
  Constant39/1 -> Product29/1
  Sum35/1 -> Product29/2
  Product29/1 -> Sum34/2
  Sum34/1 -> [RM23_pd]
  Constant33/1 -> Product26/1
  [Lthigh_cmd_trq] -> Mux29/4
  [Lshin_cmd_trq] -> Mux29/3
  [Rthigh_cmd_trq] -> Mux29/2
  [Rshin_cmd_trq] -> Mux29/1
  [Lthigh_ctrl_trq] -> Mux14/4
  [Lshin_ctrl_trq] -> Mux14/3
  [Rthigh_ctrl_trq] -> Mux14/2
  [Rshin_ctrl_trq] -> Mux14/1
  Mux15/1 -> torques/1
  Mux14/1 -> Mux15/1  "desired SEA  torques 1:4"
  Mux29/1 -> Mux15/3  "commanded motor torques 9:12"
  [RM12_des] -> Mux31/1
  [RM23_des] -> Mux31/2
  [LM12_des] -> Mux31/3
  [LM23_des] -> Mux31/4
  Mux31/1 -> Mux15/4  "desired hip/knee torques 13:16"
  [RM12_achieved] -> Mux32/1
  [RM23_achieved] -> Mux32/2
  [LM12_achieved] -> Mux32/3
  [LM23_achieved] -> Mux32/4
  Mux32/1 -> Mux15/5  "commanded hip/knee torques 17:20"
  Mux16/1 -> Mux15/6  "virtual hip/knee limit torques 21:24"
  [RKneeStop] -> Mux16/1
  [RHipStop] -> Mux16/2
  [LKneeStop] -> Mux16/3
  [LHipStop] -> Mux16/4
  [LtauF] -> Mux19/4
  [LtauB] -> Mux19/3
  [RtauF] -> Mux19/2
  [RtauB] -> Mux19/1
  Mux19/1 -> Mux15/2  "measured SEA  torques 5:8"
  [RLLoad] -> Mux28/1
  [LLLoad] -> Mux28/2
  Mux28/1 -> Mux15/7  "Est. Leg Load 25:26"
  [LLceHFL] -> Mux42/3  "lce [lopt]"
  [LFmHFL] -> Mux42/2  "F_mtu"
  [LStimHFL] -> Mux42/5  "STIM"
  [LVceHFL] -> Mux42/4  "vce [lopt]"
  [LActHFL] -> Mux42/6  "ACT"
  [LrHFL] -> Mux42/7  "moment arm"
  [LLceGLU] -> Mux41/3  "lce [lopt]"
  [LFmGLU] -> Mux41/2  "F_mtu"
  [LStimGLU] -> Mux41/5  "STIM"
  [LVceGLU] -> Mux41/4  "vce [lopt]"
  [LActGLU] -> Mux41/6  "ACT"
  [LrGLU] -> Mux41/7  "moment arm"
  [LLceHAM] -> Mux43/3  "lce [lopt]"
  [LFmHAM] -> Mux43/2  "F_mtu"
  [LStimHAM] -> Mux43/5  "STIM"
  [LVceHAM] -> Mux43/4  "vce [lopt]"
  [LActHAM] -> Mux43/6  "ACT"
  [LrHAMh] -> Mux43/7  "rh"
  [LrHAMk] -> Mux43/8  "rk"
  [LLceRF] -> Mux44/3  "lce [lopt]"
  [LFmRF] -> Mux44/2  "F_mtu"
  [LStimRF] -> Mux44/5  "STIM"
  [LVceRF] -> Mux44/4  "vce [lopt]"
  [LActRF] -> Mux44/6  "ACT"
  [LrRFh] -> Mux44/7  "rh"
  [LrRFk] -> Mux44/8  "rk"
  [LLceVAS] -> Mux40/3  "lce [lopt]"
  [LFmVAS] -> Mux40/2  "F_mtu"
  [LStimVAS] -> Mux40/5  "STIM"
  [LVceVAS] -> Mux40/4  "vce [lopt]"
  [LActVAS] -> Mux40/6  "ACT"
  [LrVAS] -> Mux40/7  "r"
  [LLceBFSH] -> Mux39/3  "lce [lopt]"
  [LFmBFSH] -> Mux39/2  "F_mtu"
  [LStimBFSH] -> Mux39/5  "STIM"
  [LVceBFSH] -> Mux39/4  "vce [lopt]"
  [LActBFSH] -> Mux39/6  "ACT"
  [LrBFSH] -> Mux39/7  "r"
  Mux43/1 -> Mux35/3  "HAM 15:22"
  Mux41/1 -> Mux35/2  "GLU 8:14"
  Mux42/1 -> Mux35/1  "HFL 1:7"
  Mux44/1 -> Mux35/4  "RF 23:30"
  Mux40/1 -> Mux35/5  "VAS 31:37"
  Mux39/1 -> Mux35/6  "BFSH 38:44"
  Mux35/1 -> L_muscle_states/1
  [LLmtuHFL] -> Mux42/1  "L_mtu"
  [LLmtuGLU] -> Mux41/1  "L_mtu"
  [LLmtuHAM] -> Mux43/1  "L_mtu"
  [LLmtuRF] -> Mux44/1  "L_mtu"
  [LLmtuVAS] -> Mux40/1  "L_mtu"
  [LLmtuHFL] -> Mux39/1  "L_mtu"
  [RLceHFL] -> Mux36/3  "lce [lopt]"
  [RFmHFL] -> Mux36/2  "F_mtu"
  [RStimHFL] -> Mux36/5  "STIM"
  [RVceHFL] -> Mux36/4  "vce [lopt]"
  [RActHFL] -> Mux36/6  "ACT"
  [RrHFL] -> Mux36/7  "moment arm"
  [RLceGLU] -> Mux34/3  "lce [lopt]"
  [RFmGLU] -> Mux34/2  "F_mtu"
  [RStimGLU] -> Mux34/5  "STIM"
  [RVceGLU] -> Mux34/4  "vce [lopt]"
  [RActGLU] -> Mux34/6  "ACT"
  [RrGLU] -> Mux34/7  "moment arm"
  [RLceHAM] -> Mux37/3  "lce [lopt]"
  [RFmHAM] -> Mux37/2  "F_mtu"
  [RStimHAM] -> Mux37/5  "STIM"
  [RVceHAM] -> Mux37/4  "vce [lopt]"
  [RActHAM] -> Mux37/6  "ACT"
  [RrHAMh] -> Mux37/7  "rh"
  [RrHAMk] -> Mux37/8  "rk"
  [RLceRF] -> Mux38/3  "lce [lopt]"
  [RFmRF] -> Mux38/2  "F_mtu"
  [RStimRF] -> Mux38/5  "STIM"
  [RVceRF] -> Mux38/4  "vce [lopt]"
  [RActRF] -> Mux38/6  "ACT"
  [RrRFh] -> Mux38/7  "rh"
  [RrRFk] -> Mux38/8  "rk"
  [RLceVAS] -> Mux33/3  "lce [lopt]"
  [RFmVAS] -> Mux33/2  "F_mtu"
  [RStimVAS] -> Mux33/5  "STIM"
  [RVceVAS] -> Mux33/4  "vce [lopt]"
  [RActVAS] -> Mux33/6  "ACT"
  [RrVAS] -> Mux33/7  "r"
  [RLceBFSH] -> Mux46/3  "lce [lopt]"
  [RFmBFSH] -> Mux46/2  "F_mtu"
  [RStimBFSH] -> Mux46/5  "STIM"
  [RVceBFSH] -> Mux46/4  "vce [lopt]"
  [RActBFSH] -> Mux46/6  "ACT"
  [RrBFSH] -> Mux46/7  "r"
  Mux37/1 -> Mux45/3  "HAM 15:22"
  Mux34/1 -> Mux45/2  "GLU 8:14"
  Mux36/1 -> Mux45/1  "HFL 1:7"
  Mux38/1 -> Mux45/4  "RF 23:30"
  Mux33/1 -> Mux45/5  "VAS 31:37"
  Mux46/1 -> Mux45/6  "BFSH 38:44"
  Mux45/1 -> R_muscle_states/1
  [RLmtuHFL] -> Mux36/1  "L_mtu"
  [RLmtuGLU] -> Mux34/1  "L_mtu"
  [RLmtuHAM] -> Mux37/1  "L_mtu"
  [RLmtuRF] -> Mux38/1  "L_mtu"
  [RLmtuVAS] -> Mux33/1  "L_mtu"
  [RLmtuHFL] -> Mux46/1  "L_mtu"
  [Lalpha] -> Mux47/2  "2"
  [Lalpha_tgt] -> Mux47/3  "3"
  [Ralpha] -> Mux47/4  "4"
  [Ralpha_tgt] -> Mux47/5  "5"
  [Lphi12] -> Mux47/9  "9"
  [Lphi23] -> Mux47/8  "8"
  [Rphi12] -> Mux47/11  "11"
  [Rphi23] -> Mux47/10  "10"
  [theta] -> Mux47/1  "1"
  [LLength] -> Mux47/6  "6"
  [RLength] -> Mux47/7  "7"
  Mux47/1 -> virtual_kinematics/1
  escape/1 -> Terminator25/1
  GRFy/1 -> Terminator26/1
  torques/1 -> Terminator13/1
  L_muscle_states/1 -> Terminator14/1
  R_muscle_states/1 -> Terminator15/1
  Constant40/1 -> Mux47/12  "12"
  Constant41/1 -> Mux47/13  "13"
  Constant42/1 -> Mux47/14  "14"
  Constant43/1 -> Mux47/15  "15"
  [Ldphi23] -> Mux47/16  "16"
  [Ldphi12] -> Mux47/17  "17"
  [Rdphi23] -> Mux47/18  "18"
  [Rdphi12] -> Mux47/19  "19"
  virtual_kinematics/1 -> Terminator16/1
  dq/1 -> Terminator17/1
  q/1 -> Terminator18/1
  Demux1/1 -> [LM12_des], L Torque/1(tau12_des [Nm])
  Demux1/2 -> [LM23_des], L Torque/2(tau23_des [Nm])
  Constant44/1 -> Mux48/1
  Constant45/1 -> Mux48/2
  Constant52/1 -> Mux48/3
  Constant53/1 -> Mux48/4
  Constant46/1 -> Mux48/5
  Constant47/1 -> Mux48/6
  Mux48/1 -> manual_switches/1
  manual_switches/1 -> Terminator19/1
  Constant50/1 -> Data Type Conversion2/1
  Constant51/1 -> Data Type Conversion3/1
  Mux49/1 -> splay angle2/1, knee angle2/1
  From260/1 -> Mux49/2
  From261/1 -> Mux49/1
  knee angle2/1 -> Goto135/1, Goto137/1
  From262/1 -> Sum37/2
  From267/1 -> Sum37/1
  Sum37/1 -> Gain6/1, Goto134/1
  Gain6/1 -> Goto136/1, Goto138/1
  splay angle2/1 -> Goto133/1
  Mux50/1 -> splay angle3/1, knee angle3/1
  From263/1 -> Mux50/2
  From264/1 -> Mux50/1
  knee angle3/1 -> Goto141/1, Goto143/1
  From265/1 -> Sum36/2
  From266/1 -> Sum36/1
  Sum36/1 -> Goto140/1, Gain7/1
  Gain7/1 -> Goto142/1, Goto144/1
  splay angle3/1 -> Goto139/1
  Constant48/1 -> Mux48/7
  Constant49/1 -> Mux48/8
  [Lphi12] -> L Knee Joint Limits2/1(phi [rad]1), VAS Link2/1(phi23 [rad]), RF Link2/2(phi23 [rad]), HAM Link2/2(phi23 [rad]), L BFSH Link2/1(phi23 [rad])
  [LStimHAM] -> HAM/1(STIM)
  HAM/1(Fmtc) -> Product45/1, Product44/1, [LFmHAM]
  HAM/2(Lce) -> R HAM Muscle Spindles5/1
  HFL/1(Fmtc) -> Product43/2, [LFmHFL]
  HFL/2(Lce) -> L HFL Muscle Spindles8/1
  [LStimHFL] -> HFL/1(STIM)
  GLU/1(Fmtc) -> Product42/1, [LFmGLU]
  [LStimGLU] -> GLU/1(STIM)
  Sum44/1 -> [LM23]
  [Ldphi12] -> L Knee Joint Limits2/2(dphi [rad/s]1)
  VAS Link2/1(lmtu [m]) -> [LLmtuVAS], VAS/2(lmtc [m])
  HAM Link2/1(lmtu [m]) -> [LLmtuHAM], HAM/2(lmtc [m])
  HAM Link2/2(lever34 [m]) -> Product44/2, [LrHAMh]
  HAM Link2/3(lever23 [m]) -> Product45/2, [LrHAMk]
  Sum50/1 -> Sum43/1
  [Lphi23] -> L Hip Joint Limits2/1(phi [rad]1), HFL Link2/1(phi34 [rad]), GLU Link2/1(phi34 [rad]), RF Link2/1(phi34 [rad]), HAM Link2/1(phi34 [rad])
  VAS/4(A) -> [LActVAS]
  VAS/1(Fmtc) -> Product40/2, [LFmVAS]
  Sum38/1 -> [LM12]
  L Knee Joint Limits2/1(M_stop [Nm]1) -> Sum38/1, [LKneeStop]
  Sum51/1 -> Sum38/2
  VAS Link2/2(lever [m]) -> [LrVAS], Product40/1
  Sum49/1 -> Sum51/1
  HAM/4(A) -> [LActHAM]
  Product44/1 -> Sum50/2
  Product42/1 -> Sum50/1
  GLU Link2/1(lmtu [m]) -> [LLmtuGLU], GLU/2(lmtc [m])
  GLU Link2/2(lever [m]) -> Product42/2, [LrGLU]
  GLU/4(A) -> [LActGLU]
  [Ldphi23] -> L Hip Joint Limits2/2(dphi [rad/s]1)
  L Hip Joint Limits2/1(M_stop [Nm]1) -> [LHipStop], Sum44/1
  Sum43/1 -> Sum44/2
  HFL Link2/1(lmtu [m]) -> [LLmtuHFL], HFL/2(lmtc [m])
  HFL/4(A) -> [LActHFL]
  HFL Link2/2(lever [m]) -> Product43/1, [LrHFL]
  [LStimVAS] -> VAS/1(STIM)
  GLU/2(Lce) -> L HFL Muscle Spindles11/1
  GLU/3(Vce) -> L HFL Muscle Spindles10/1
  HAM/3(Vce) -> R HAM Muscle Spindles16/1
  VAS/3(Vce) -> L RF Muscle Spindles14/1
  VAS/2(Lce) -> L RF Muscle Spindles12/1
  HFL/3(Vce) -> L HFL Muscle Spindles9/1
  RF/4(A) -> [LActRF]
  RF/3(Vce) -> L RF Muscle Spindles10/1
  RF/2(Lce) -> L RF Muscle Spindles8/1
  RF Link2/1(lmtu [m]) -> [LLmtuRF], RF/2(lmtc [m])
  RF Link2/2(lever34 [m]) -> Product41/1, [LrRFh]
  RF Link2/3(lever23 [m]) -> Product32/1, [LrRFk]
  [LStimRF] -> RF/1(STIM)
  Product43/1 -> Sum40/1
  Product41/1 -> Sum40/2
  Product32/1 -> Sum45/2
  Sum45/1 -> Sum51/2
  Product40/1 -> Sum45/1
  [LStimBFSH] -> L BFSH1/1(STIM)
  L BFSH Link2/1(lmtu [m]) -> [LLmtuBFSH], L BFSH1/2(lmtc [m])
  L BFSH Link2/2(lever [m]) -> [LrBFSH], Product36/2
  L BFSH1/4(A) -> [LActBFSH]
  L BFSH1/2(Lce) -> R HAM Muscle Spindles15/1
  L BFSH1/3(Vce) -> R HAM Muscle Spindles10/1
  Product36/1 -> Sum49/2
  Product45/1 -> Sum49/1
  L HFL Muscle Spindles9/1 -> [LVceHFL]
  L HFL Muscle Spindles10/1 -> [LVceGLU]
  L HFL Muscle Spindles11/1 -> [LLceGLU]
  L RF Muscle Spindles14/1 -> [LVceVAS]
  RF/1(Fmtc) -> Product41/2, Product32/2, [LFmRF]
  L BFSH1/1(Fmtc) -> Product36/1, [LFmBFSH]
  L HFL Muscle Spindles8/1 -> [LLceHFL]
  R HAM Muscle Spindles5/1 -> [LLceHAM]
  R HAM Muscle Spindles16/1 -> [LVceHAM]
  L RF Muscle Spindles8/1 -> [LLceRF]
  L RF Muscle Spindles10/1 -> [LVceRF]
  R HAM Muscle Spindles15/1 -> [LLceBFSH]
  R HAM Muscle Spindles10/1 -> [LVceBFSH]
  L RF Muscle Spindles12/1 -> [LLceVAS]
  [Rphi12] -> L Knee Joint Limits3/1(phi [rad]1), VAS Link3/1(phi23 [rad]), HAM Link3/2(phi23 [rad]), RF Link3/2(phi23 [rad]), L BFSH Link3/1(phi23 [rad])
  [RStimHAM] -> HAM1/1(STIM)
  HAM1/1(Fmtc) -> Product39/1, Product38/1, [RFmHAM]
  HAM1/2(Lce) -> R HAM Muscle Spindles11/1
  HFL1/1(Fmtc) -> Product37/2, [RFmHFL]
  HFL1/2(Lce) -> L HFL Muscle Spindles12/1
  [RStimHFL] -> HFL1/1(STIM)
  GLU1/1(Fmtc) -> Product35/1, [RFmGLU]
  [RStimGLU] -> GLU1/1(STIM)
  Sum41/1 -> [RM23]
  [Rdphi12] -> L Knee Joint Limits3/2(dphi [rad/s]1)
  VAS Link3/1(lmtu [m]) -> [RLmtuVAS], VAS1/2(lmtc [m])
  HAM Link3/1(lmtu [m]) -> [RLmtuHAM], HAM1/2(lmtc [m])
  HAM Link3/2(lever34 [m]) -> Product38/2, [RrHAMh]
  HAM Link3/3(lever23 [m]) -> Product39/2, [RrHAMk]
  Sum47/1 -> Sum39/1
  [Rphi23] -> L Hip Joint Limits3/1(phi [rad]1), HFL Link3/1(phi34 [rad]), GLU Link3/1(phi34 [rad]), RF Link3/1(phi34 [rad]), HAM Link3/1(phi34 [rad])
  VAS1/4(A) -> [RActVAS]
  VAS1/1(Fmtc) -> Product33/2, [RFmVAS]
  Sum52/1 -> [RM12]
  L Knee Joint Limits3/1(M_stop [Nm]1) -> Sum52/1, [RKneeStop]
  Sum48/1 -> Sum52/2
  VAS Link3/2(lever [m]) -> [RrVAS], Product33/1
  Sum46/1 -> Sum48/1
  HAM1/4(A) -> [RActHAM]
  Product38/1 -> Sum47/2
  Product35/1 -> Sum47/1
  GLU Link3/1(lmtu [m]) -> [RLmtuGLU], GLU1/2(lmtc [m])
  GLU Link3/2(lever [m]) -> Product35/2, [RrGLU]
  GLU1/4(A) -> [RActGLU]
  [Rdphi23] -> L Hip Joint Limits3/2(dphi [rad/s]1)
  L Hip Joint Limits3/1(M_stop [Nm]1) -> [RHipStop], Sum41/1
  Sum39/1 -> Sum41/2
  HFL Link3/1(lmtu [m]) -> [RLmtuHFL], HFL1/2(lmtc [m])
  HFL1/4(A) -> [RActHFL]
  HFL Link3/2(lever [m]) -> Product37/1, [RrHFL]
  [RStimVAS] -> VAS1/1(STIM)
  GLU1/2(Lce) -> L HFL Muscle Spindles15/1
  GLU1/3(Vce) -> L HFL Muscle Spindles14/1
  HAM1/3(Vce) -> R HAM Muscle Spindles9/1
  VAS1/3(Vce) -> L RF Muscle Spindles15/1
  VAS1/2(Lce) -> L RF Muscle Spindles13/1
  HFL1/3(Vce) -> L HFL Muscle Spindles13/1
  RF1/4(A) -> [RActRF]
  RF1/3(Vce) -> L RF Muscle Spindles11/1
  RF1/2(Lce) -> L RF Muscle Spindles9/1
  RF Link3/1(lmtu [m]) -> [RLmtuRF], RF1/2(lmtc [m])
  RF Link3/2(lever34 [m]) -> Product34/1, [RrRFh]
  RF Link3/3(lever23 [m]) -> [RrRFk], Product30/1
  [RStimRF] -> RF1/1(STIM)
  Sum53/1 -> Sum39/2
  Product37/1 -> Sum53/1
  Product34/1 -> Sum53/2
  Product30/1 -> Sum42/2
  Sum42/1 -> Sum48/2
  Product33/1 -> Sum42/1
  [RStimBFSH] -> L BFSH2/1(STIM)
  L BFSH Link3/1(lmtu [m]) -> [RLmtuBFSH], L BFSH2/2(lmtc [m])
  L BFSH Link3/2(lever [m]) -> [RrBFSH], Product31/2
  L BFSH2/4(A) -> [RActBFSH]
  L BFSH2/2(Lce) -> R HAM Muscle Spindles8/1
  L BFSH2/3(Vce) -> R HAM Muscle Spindles7/1
  Product31/1 -> Sum46/2
  Product39/1 -> Sum46/1
  L HFL Muscle Spindles13/1 -> [RVceHFL]
  L HFL Muscle Spindles14/1 -> [RVceGLU]
  L HFL Muscle Spindles15/1 -> [RLceGLU]
  L RF Muscle Spindles15/1 -> [RVceVAS]
  RF1/1(Fmtc) -> Product34/2, Product30/2, [RFmRF]
  L BFSH2/1(Fmtc) -> Product31/1, [RFmBFSH]
  L HFL Muscle Spindles12/1 -> [RLceHFL]
  R HAM Muscle Spindles11/1 -> [RLceHAM]
  R HAM Muscle Spindles9/1 -> [RVceHAM]
  L RF Muscle Spindles9/1 -> [RLceRF]
  L RF Muscle Spindles11/1 -> [RVceRF]
  R HAM Muscle Spindles8/1 -> [RLceBFSH]
  R HAM Muscle Spindles7/1 -> [RVceBFSH]
  L RF Muscle Spindles13/1 -> [RLceVAS]
  Sum40/1 -> Sum43/2
